simulink library "bh_6dof_LIBRARY"  (R2016a)
settings: Solver=VariableStepAuto  StartTime=0.0  StopTime=10.0  RelTol=1e-3
undefined symbols (not defined in the file): mot_1_volts, mot_2_volts, mot_3_volts, mot_4_volts, P_veh
libraries: simulink_extras x3, bh_6dof_LIBRARY x1
settings Model: Creator=bhorton  LastModifiedBy=bhorton
settings DataIOCC: LimitDataPoints=on
settings DebuggingCC: AllowSymbolicDim=off
settings ModelReferenceCC: PropagateSignalLabelsOutOfModel=off
settings GRTTargetCC: GeneratePreprocessorConditionals=Use local settings

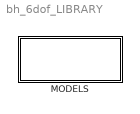
== system bh_6dof_LIBRARY ==
  MODELS : Subsystem

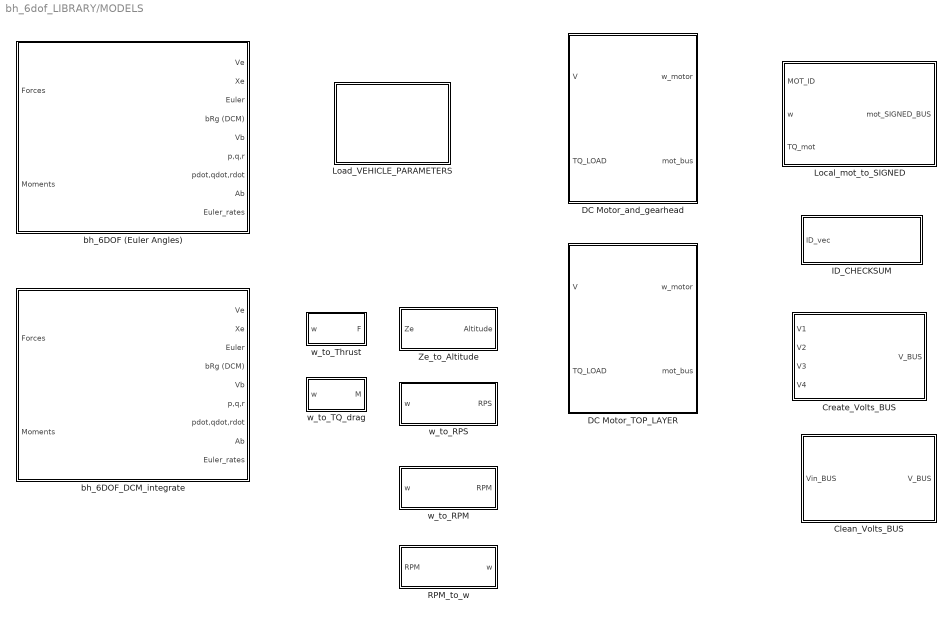
== system bh_6dof_LIBRARY/MODELS ==
  Clean_Volts_BUS : Subsystem  mask{v_min=0, v_max=7}
      mask prompts: v_min "V minimun (volts)"; v_max "V maximum (volts)"
      mask Display: fprintf('CLEAN \n\n VOLTS BUS \n\n Vmin = %.2f \n Vmax = %.2f',v_min, v_max);
  Create_Volts_BUS : Subsystem  mask{v_min=0, v_max=7}
      mask prompts: v_min "V minimun (volts)"; v_max "V maximum (volts)"
      mask Display: fprintf('VOLTS BUS \n\n Vmin = %.2f \n Vmax = %.2f',v_min, v_max);
  DC Motor_TOP_LAYER : Subsystem  mask(DC motor){P_mot_S=struct('ID',0,'Ka',1,'b',1,'I',1,'R',1,'L',1,'Ke',1)}
      mask prompts: P_mot_S "Enter your MOTOR param STRUCT"
      mask help: DC motor
      mask DialogControl Container9 Prompt: Tab
      mask Display: fprintf('DC motor\n\nID= %d',P_mot_S.ID)
  DC Motor_and_gearhead : Subsystem  mask(DC motor){K=1, B=1e-6, J=1e-7, GearRatio=1, R=1, L=1, Kb=1, ID=1}
      mask prompts: K "Torque constant (N.m/A)"; B "Viscous friction co-efficient (N.m.s)"; J "Rotor Inertia (kg.m^2)"; GearRatio "Gear ratio (w_motor/w_wheel)"; R "Armature resistance (ohms)"; L "Armature Inductance (Henry)"; Kb "Back Emf constant (V.sec/rad)"; ID "Motor_ID  (#1 to #4)"
      mask help: DC motor
      mask Display: disp('DC motor')
  ID_CHECKSUM : Subsystem
      mask Display: fprintf('ID\nChecksum')
  Load_VEHICLE_PARAMETERS : Subsystem
      settings: OpenFcn=bh_quad_params
      mask Display: disp('Double click\nto\nLOAD\nvehicle \n parameters')
  Local_mot_to_SIGNED : Subsystem
  RPM_to_w : Subsystem
      mask Display: fprintf('RPM\nto\nw(rad/sec)')
  Ze_to_Altitude : Subsystem
      mask Display: fprintf('Ze \n to \n ALTITUDE');
  bh_6DOF (Euler Angles) : Subsystem  mask(bh_6DOF EoM (Body Axis)){inertia_0=P_veh.I, mass_0=P_veh.mass, xme_0=P_veh.Xe_init, Vm_0=P_veh.Vb_init, pm_0=P_veh.wb_init, eul_0=P_veh.eul_init}
      mask prompts: inertia_0 "Vehicle Inertia, [kg.m^2]"; mass_0 "Vehicle Mass, [kg]"; xme_0 "Initial position in inertial axes [Xe,Ye,Ze], [m]"; Vm_0 "Initial velocity in body axes [U,v,w], [m/sec]"; pm_0 "Initial body rotation rates [p,q,r], [rad/sec]"; eul_0 "Initial Euler orientation [yaw, pitch, roll], [rad]"
      mask DialogControl DescTextVar Prompt: Implementation of a 6-DOF rigid body equations of motion.
      mask DialogControl Control16 Prompt: Euler angles are used to describe angular pose.
      mask DialogControl Control22 Prompt: The co-ordinate transformation that converts the components of a
      mask DialogControl Control23 Prompt: G-frame vector into its components in the B-frame, is:
      mask DialogControl Control24 Prompt: vb = pR3X(psi) * pR2Y(theta) * pR1Z(phi) * vg
      mask DialogControl Control25 Prompt: vb = bRg * vg
      mask DialogControl Control53 Prompt: You can READ more about PASSIVE rotations, HERE.
      mask DialogControl Control53 Callback: winopen('CONCEPT_PASSIVE_rotations.pdf')
      mask DialogControl Control26 Prompt: To actively reposition (ie: rotate) a B-frame that is initially coincident
      mask DialogControl Control27 Prompt: with the inertial G-frame, into a new pose, we would:
      mask DialogControl Control28 Prompt: vg = inv(pR1Z(phi)) * inv(pR2Y(theta)) * inv(pR3X(psi)) * vb
      mask DialogControl Control30 Prompt: If we define:    aR( ) == inv( pR()  ),  then we can write the above as:
      mask DialogControl Control32 Prompt: vg = aR1Z(phi) * aR2Y(theta) * aR3(psi) * vb
      mask DialogControl Control40 Prompt: You can READ more about ACTIVE rotations, HERE.
      mask DialogControl Control40 Callback: winopen('CONCEPT_ACTIVE_rotations.pdf')
      mask DialogControl Control11 Prompt: ATTENTION:  note the order of the angles in the list above.
      mask DialogControl Control12 Prompt: This is DIFFERENT to the order used in the Aerospace blockset.
      mask DialogControl Control6 Prompt: In this EULER angle implementation we define the
      mask DialogControl Control7 Prompt: following sequence that rotates a G-frame
      mask DialogControl Control8 Prompt: into a B-frame:
      mask DialogControl Control9_copy Prompt: 1.)  R1Z  : a local rotation about the Z axis by phi, (YAW)
      mask DialogControl Control9_copy_copy Prompt: 2.)  R2Y  : a local rotation about the Y axis by theta, (PITCH)
      mask DialogControl Control17 Prompt: 3.)  R3X  : a local rotation about the X axis by psi, (ROLL)
      mask DialogControl Control18 Prompt: The translational Rigid body Equations of motion are:
      mask DialogControl Control20 Prompt: The rotational Rigid body Equations of motion are
      mask Display:
      | port_label('input',1,'{{Fb_{xyz}} (N)}','texmode','on');
      | port_label('input',2,'{{Mb_{xyz}} (N-m)}','texmode','on');
      | port_label('output',1,'{V_e (m/s)}','texmode','on');
      | port_label('output',2,'{X_e (m)}','texmode','on');
      | port_label('output',3,'{\Phi_{Z1} \theta_{Y2} \Psi_{X3} (rad)}','texmode','on');
      | port_label('output',4,'{DCM bRg }','texmode','on');
      | port_label('output',5,'{V_b (m/s)}','texmode','on');
      | port_label('output',6,'{{\omega_b (rad/s)}}','texmode','on');
      | port_label('output',7,'{{d\omega_b/dt}}','texmode','on');
      | port_label('output',8,'{A_b (m/s^2)}','texmode','on');
      | port_label('output',9,'{d\Phi_{Z1} d\theta_{Y2} d\Psi_{X3} (rad/sec)}','texmode','on');
      | 
      | text(0.5,0.7248,'Body\nEuler Angles','horizontalAlignment','center')
      | text(0.5,0.3112,'Fixed\nMass','horizontalAlignment','center')
  bh_6DOF_DCM_integrate : Subsystem  mask(bh_6DOF EoM (Body Axis) DCM approach){inertia_0=P_veh.I, mass_0=P_veh.mass, xme_0=P_veh.Xe_init, Vm_0=P_veh.Vb_init, pm_0=P_veh.wb_init, eul_0=P_veh.eul_init}
      mask prompts: inertia_0 "Vehicle Inertia, [kg.m^2]"; mass_0 "Vehicle Mass, [kg]"; xme_0 "Initial position in inertial axes [Xe,Ye,Ze], [m]"; Vm_0 "Initial velocity in body axes [U,v,w], [m/sec]"; pm_0 "Initial body rotation rates [p,q,r], [rad/sec]"; eul_0 "Initial Euler orientation [yaw, pitch, roll], [rad]"
      mask DialogControl DescTextVar Prompt: Implementation of a 6-DOF rigid body equations of motion.
      mask DialogControl Control16 Prompt: Euler angles are used to describe angular pose. We integrate the DCM derivative to calculate the Euler angles.
      mask DialogControl Control22 Prompt: The co-ordinate transformation that converts the components of a
      mask DialogControl Control23 Prompt: G-frame vector into its components in the B-frame, is:
      mask DialogControl Control24 Prompt: vb = pR3X(psi) * pR2Y(theta) * pR1Z(phi) * vg
      mask DialogControl Control25 Prompt: vb = bRg * vg
      mask DialogControl Control53 Prompt: You can READ more about PASSIVE rotations, HERE.
      mask DialogControl Control53 Callback: winopen('CONCEPT_PASSIVE_rotations.pdf')
      mask DialogControl Control26 Prompt: To actively reposition (ie: rotate) a B-frame that is initially coincident
      mask DialogControl Control27 Prompt: with the inertial G-frame, into a new pose, we would:
      mask DialogControl Control28 Prompt: vg = inv(pR1Z(phi)) * inv(pR2Y(theta)) * inv(pR3X(psi)) * vb
      mask DialogControl Control30 Prompt: If we define:    aR( ) == inv( pR()  ),  then we can write the above as:
      mask DialogControl Control32 Prompt: vg = aR1Z(phi) * aR2Y(theta) * aR3(psi) * vb
      mask DialogControl Control40 Prompt: You can READ more about ACTIVE rotations, HERE.
      mask DialogControl Control40 Callback: winopen('CONCEPT_ACTIVE_rotations.pdf')
      mask DialogControl Control11 Prompt: ATTENTION:  note the order of the angles in the list above.
      mask DialogControl Control12 Prompt: This is DIFFERENT to the order used in the Aerospace blockset.
      mask DialogControl Control6 Prompt: In this EULER angle implementation we define the
      mask DialogControl Control7 Prompt: following sequence that rotates a G-frame
      mask DialogControl Control8 Prompt: into a B-frame:
      mask DialogControl Control9_copy Prompt: 1.)  R1Z  : a local rotation about the Z axis by phi, (YAW)
      mask DialogControl Control9_copy_copy Prompt: 2.)  R2Y  : a local rotation about the Y axis by theta, (PITCH)
      mask DialogControl Control17 Prompt: 3.)  R3X  : a local rotation about the X axis by psi, (ROLL)
      mask DialogControl Control18 Prompt: The translational Rigid body Equations of motion are:
      mask DialogControl Control20 Prompt: The rotational Rigid body Equations of motion are
      mask Display:
      | port_label('input',1,'{{Fb_{xyz}} (N)}','texmode','on');
      | port_label('input',2,'{{Mb_{xyz}} (N-m)}','texmode','on');
      | port_label('output',1,'{V_e (m/s)}','texmode','on');
      | port_label('output',2,'{X_e (m)}','texmode','on');
      | port_label('output',3,'{\Phi_{Z1} \theta_{Y2} \Psi_{X3} (rad)}','texmode','on');
      | port_label('output',4,'{DCM bRg }','texmode','on');
      | port_label('output',5,'{V_b (m/s)}','texmode','on');
      | port_label('output',6,'{{\omega_b (rad/s)}}','texmode','on');
      | port_label('output',7,'{{d\omega_b/dt}}','texmode','on');
      | port_label('output',8,'{A_b (m/s^2)}','texmode','on');
      | port_label('output',9,'{d\Phi_{Z1} d\theta_{Y2} d\Psi_{X3} (rad/sec)}','texmode','on');
      | 
      | text(0.5,0.7248,'DCM\nintegration','horizontalAlignment','center')
      | 
      | text(0.5,0.3112,'Fixed\nMass','horizontalAlignment','center')
  w_to_RPM : Subsystem
      mask Display: fprintf('w(rad/sec)\nto\nRPM')
  w_to_RPS : Subsystem
      mask Display: fprintf('w(rad/sec)\nto\nRPS')
  w_to_TQ_drag : Subsystem  mask(w_to_TQdrag){k=0}
      mask prompts: k "k (N/ ( rad/sec)^2 )"
      mask help:
      | Convert angular speed w(rad/sec) into drag TORQUE,  M (N.m).
      | A simple quadratic rule is used:
      |
      | M = k * w^2
      settings: AttributesFormatString=k = %<k>
  w_to_Thrust : Subsystem  mask(w_to_thrust){k=0}
      mask prompts: k "k (N/ ( rad/sec)^2 )"
      mask help:
      | Convert angular speed w(rad/sec) into lift thrust F (N).
      | A simple quadratic rule is used:
      |
      | F = k * w^2
      settings: AttributesFormatString=k = %<k>

== system bh_6dof_LIBRARY/MODELS/Clean_Volts_BUS ==
  Vin_BUS : Inport
  Bus Assignment : BusAssignment  AssignedSignals=mot_1_volts,mot_2_volts,mot_3_volts,mot_4_volts
  Bus Selector : BusSelector  OutputSignals=mot_1_volts,mot_2_volts,mot_3_volts,mot_4_volts
  Saturation{4..7} (4 alike) : Saturate  UpperLimit=v_max  LowerLimit=v_min
  V_BUS : Outport
  wires:
  Bus Selector/1 -> Saturation4/1  "<mot_1_volts>"
  Bus Selector/2 -> Saturation5/1  "<mot_2_volts>"
  Bus Selector/3 -> Saturation6/1  "<mot_3_volts>"
  Bus Selector/4 -> Saturation7/1  "<mot_4_volts>"
  Vin_BUS/1 -> Bus Assignment/1, Bus Selector/1
  Saturation4/1 -> Bus Assignment/2
  Saturation7/1 -> Bus Assignment/5
  Saturation6/1 -> Bus Assignment/4
  Saturation5/1 -> Bus Assignment/3
  Bus Assignment/1 -> V_BUS/1

== system bh_6dof_LIBRARY/MODELS/Create_Volts_BUS ==
  V1 : Inport
  V2 : Inport  Port=2
  V3 : Inport  Port=3
  V4 : Inport  Port=4
  Bus Creator : BusCreator  Inputs=4
  Saturation{,1..3} (4 alike) : Saturate  UpperLimit=v_max  LowerLimit=v_min
  V_BUS : Outport
  wires:
  Bus Creator/1 -> V_BUS/1
  Saturation/1 -> Bus Creator/1  "mot_1_volts"
  Saturation3/1 -> Bus Creator/4  "mot_4_volts"
  Saturation2/1 -> Bus Creator/3  "mot_3_volts"
  Saturation1/1 -> Bus Creator/2  "mot_2_volts"
  V1/1 -> Saturation/1
  V2/1 -> Saturation1/1
  V3/1 -> Saturation2/1
  V4/1 -> Saturation3/1

== system bh_6dof_LIBRARY/MODELS/DC Motor_TOP_LAYER ==
  V : Inport
  TQ_LOAD : Inport  Port=2
  DC Motor_and_gearhead : bh_6dof_LIBRARY/MODELS/DC Motor_and_gearhead  K=P_mot_S.Ka  B=P_mot_S.b  J=P_mot_S.I  R=P_mot_S.R  L=P_mot_S.L  Kb=P_mot_S.Ke  ID=P_mot_S.ID
  w_motor : Outport
  mot_bus : Outport  Port=2
  wires:
  DC Motor_and_gearhead/2 -> mot_bus/1
  DC Motor_and_gearhead/1 -> w_motor/1
  TQ_LOAD/1 -> DC Motor_and_gearhead/2
  V/1 -> DC Motor_and_gearhead/1

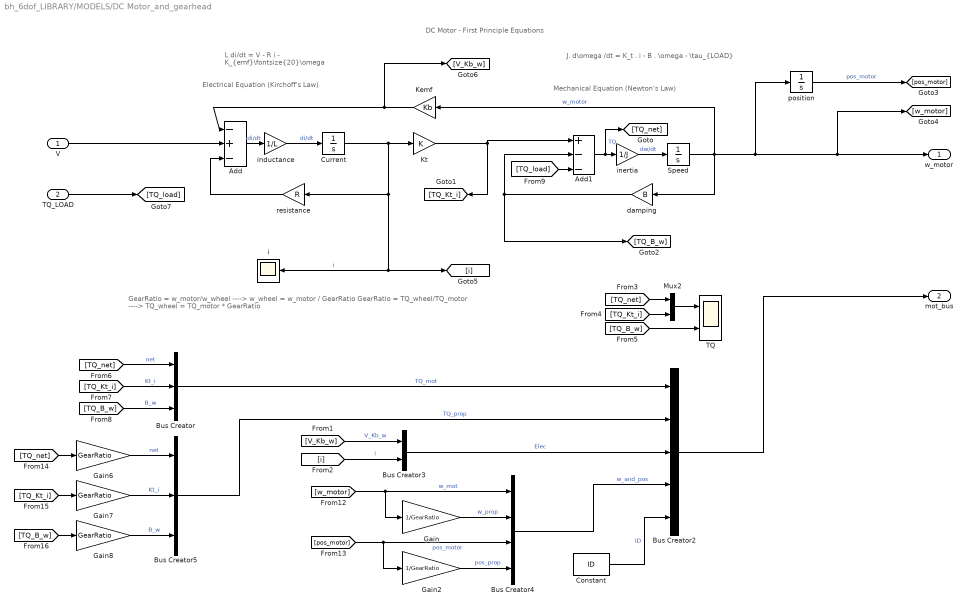
== system bh_6dof_LIBRARY/MODELS/DC Motor_and_gearhead ==
  note: GearRatio = w_motor/w_wheel    ---->   w_wheel = w_motor / GearRatio
      |
      | GearRatio = TQ_wheel/TQ_motor  ---->  TQ_wheel = TQ_motor * GearRatio
  note: Mechanical Equation
      | (Newton's Law)
  note: L di/dt = V - R i - K_{emf}\fontsize{20}\omega
  note: J. d\omega /dt = K_t . i - B . \omega - \tau_{LOAD}
  note: DC Motor - First Principle Equations
  note: Electrical Equation
      | (Kirchoff's Law)
  V : Inport
  TQ_LOAD : Inport  Port=2
  Add : Sum  Inputs=-+-
  Add1 : Sum  Inputs=+--
  Bus Creator : BusCreator  Inputs=3
  Bus Creator2 : BusCreator  Inputs=5
  Bus Creator3 : BusCreator  Inputs=2
  Bus Creator4 : BusCreator  Inputs=4
  Bus Creator5 : BusCreator  Inputs=3
  Constant : Constant  Value=ID
  Current : Integrator
  Gain : Gain  Gain=1/GearRatio
  Gain2 : Gain  Gain=1/GearRatio
  Gain6 : Gain  Gain=GearRatio
  Gain7 : Gain  Gain=GearRatio
  Gain8 : Gain  Gain=GearRatio
  Kemf : Gain  Gain=Kb
  Kt : Gain  Gain=K
  Mux2 : Mux  Inputs=2
  Speed : Integrator
  TQ : Scope  NumInputPorts=2
  damping : Gain  Gain=B
  i : Scope
  inductance : Gain  Gain=1/L
  inertia : Gain  Gain=1/J
  position : Integrator
  resistance : Gain  Gain=R
  w_motor : Outport
  mot_bus : Outport  Port=2
  wires:
  inertia/1 -> Speed/1  "dw/dt"
  damping/1 -> [TQ_B_w], Add1/2
  Kt/1 -> Add1/1, [TQ_Kt_i]
  inductance/1 -> Current/1  "di/dt"
  Speed/1 -> Kemf/1, position/1, [w_motor], w_motor/1, damping/1  "w_motor"
  Add1/1 -> [TQ_net], inertia/1  "TQ"
  Current/1 -> Kt/1, resistance/1, [i], i/1  "i"
  Add/1 -> inductance/1  "di/dt"
  resistance/1 -> Add/3
  Kemf/1 -> [V_Kb_w], Add/1
  position/1 -> [pos_motor]  "pos_motor"
  Mux2/1 -> TQ/1
  [TQ_net] -> Mux2/1
  [TQ_Kt_i] -> Mux2/2
  [TQ_B_w] -> TQ/2
  [TQ_net] -> Bus Creator/1  "net"
  [TQ_B_w] -> Bus Creator/3  "B_w"
  [TQ_Kt_i] -> Bus Creator/2  "Kt_i"
  Bus Creator/1 -> Bus Creator2/1  "TQ_mot"
  [i] -> Bus Creator3/2  "i"
  [V_Kb_w] -> Bus Creator3/1  "V_Kb_w"
  [w_motor] -> Gain/1, Bus Creator4/1  "w_mot"
  Gain/1 -> Bus Creator4/2  "w_prop"
  [pos_motor] -> Gain2/1, Bus Creator4/3  "pos_motor"
  Gain2/1 -> Bus Creator4/4  "pos_prop"
  Bus Creator5/1 -> Bus Creator2/2  "TQ_prop"
  Bus Creator4/1 -> Bus Creator2/4  "w_and_pos"
  Bus Creator3/1 -> Bus Creator2/3  "Elec"
  Bus Creator2/1 -> mot_bus/1
  [TQ_net] -> Gain6/1
  Gain6/1 -> Bus Creator5/1  "net"
  Gain8/1 -> Bus Creator5/3  "B_w"
  Gain7/1 -> Bus Creator5/2  "Kt_i"
  [TQ_Kt_i] -> Gain7/1
  [TQ_B_w] -> Gain8/1
  TQ_LOAD/1 -> [TQ_load]
  [TQ_load] -> Add1/3
  V/1 -> Add/2
  Constant/1 -> Bus Creator2/5  "ID"

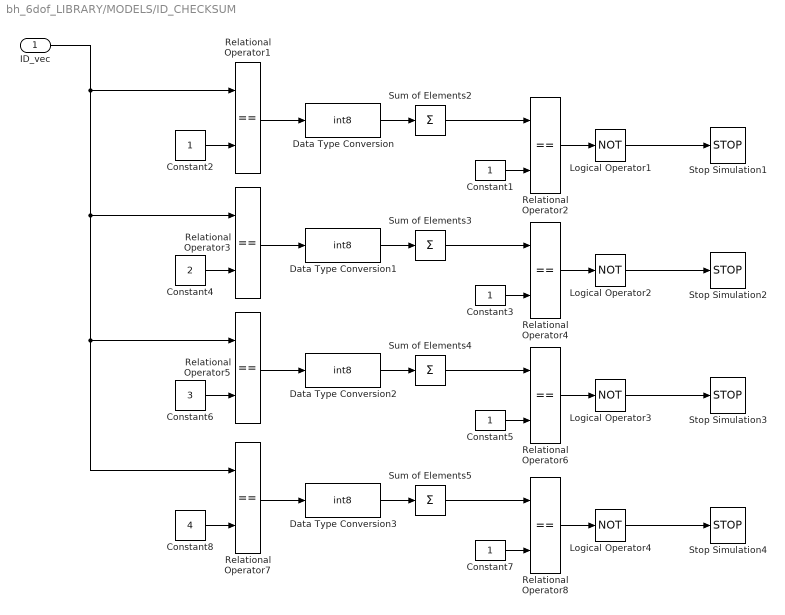
== system bh_6dof_LIBRARY/MODELS/ID_CHECKSUM ==
  ID_vec : Inport
  Constant{1..3,5,7} (5 alike) : Constant
  Constant4 : Constant  Value=2
  Constant6 : Constant  Value=3
  Constant8 : Constant  Value=4
  Data Type Conversion{,1..3} (4 alike) : DataTypeConversion  OutDataTypeStr=int8
  Logical Operator{1..4} (4 alike) : Logic  Operator=NOT  AllPortsSameDT=off  OutDataTypeStr=boolean
  Relational Operator{1..8} (8 alike) : RelationalOperator  Operator===  OutDataTypeStr=boolean
  Stop Simulation{1..4} (4 alike) : Stop
  Sum of Elements{2..5} (4 alike) : Sum  Inputs=+
  wires:
  Relational Operator1/1 -> Data Type Conversion/1
  Data Type Conversion/1 -> Sum of Elements2/1
  Sum of Elements2/1 -> Relational Operator2/1
  Constant1/1 -> Relational Operator2/2
  Relational Operator2/1 -> Logical Operator1/1
  Constant2/1 -> Relational Operator1/2
  Logical Operator1/1 -> Stop Simulation1/1
  Relational Operator3/1 -> Data Type Conversion1/1
  Data Type Conversion1/1 -> Sum of Elements3/1
  Sum of Elements3/1 -> Relational Operator4/1
  Constant3/1 -> Relational Operator4/2
  Relational Operator4/1 -> Logical Operator2/1
  Constant4/1 -> Relational Operator3/2
  Logical Operator2/1 -> Stop Simulation2/1
  Relational Operator5/1 -> Data Type Conversion2/1
  Data Type Conversion2/1 -> Sum of Elements4/1
  Sum of Elements4/1 -> Relational Operator6/1
  Constant5/1 -> Relational Operator6/2
  Relational Operator6/1 -> Logical Operator3/1
  Constant6/1 -> Relational Operator5/2
  Logical Operator3/1 -> Stop Simulation3/1
  ID_vec/1 -> Relational Operator7/1, Relational Operator5/1, Relational Operator3/1, Relational Operator1/1
  Relational Operator7/1 -> Data Type Conversion3/1
  Data Type Conversion3/1 -> Sum of Elements5/1
  Sum of Elements5/1 -> Relational Operator8/1
  Constant7/1 -> Relational Operator8/2
  Relational Operator8/1 -> Logical Operator4/1
  Constant8/1 -> Relational Operator7/2
  Logical Operator4/1 -> Stop Simulation4/1

== system bh_6dof_LIBRARY/MODELS/Load_VEHICLE_PARAMETERS ==

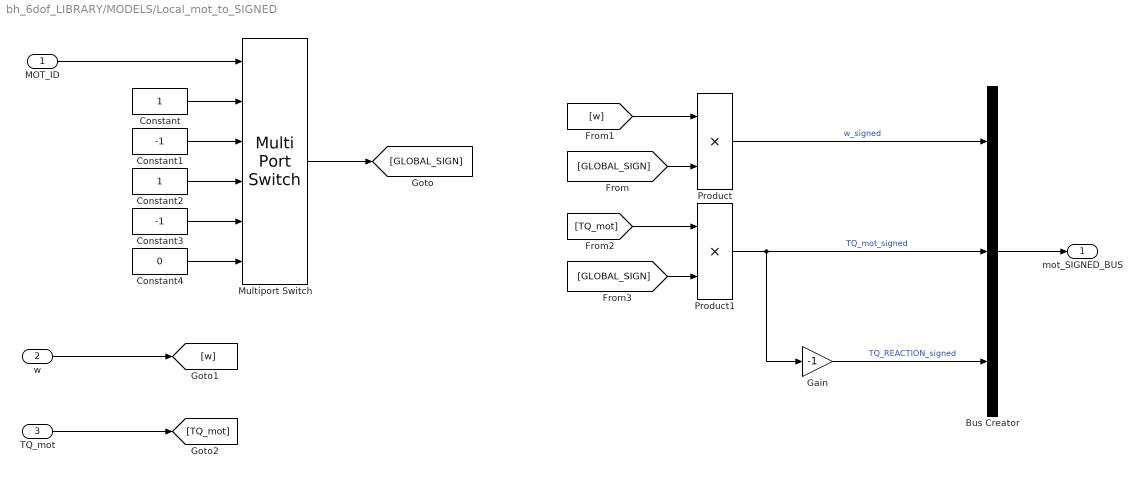
== system bh_6dof_LIBRARY/MODELS/Local_mot_to_SIGNED ==
  MOT_ID : Inport
  w : Inport  Port=2
  TQ_mot : Inport  Port=3
  Bus Creator : BusCreator  Inputs=3
  Constant : Constant
  Constant1 : Constant  Value=-1
  Constant2 : Constant
  Constant3 : Constant  Value=-1
  Constant4 : Constant  Value=0
  Gain : Gain  Gain=-1
  Multiport Switch : MultiPortSwitch  Inputs=4  DataPortForDefault=Additional data port
  Product : Product
  Product1 : Product
  mot_SIGNED_BUS : Outport
  wires:
  Constant1/1 -> Multiport Switch/3
  Constant/1 -> Multiport Switch/2
  Constant3/1 -> Multiport Switch/5
  Constant4/1 -> Multiport Switch/6
  MOT_ID/1 -> Multiport Switch/1
  Constant2/1 -> Multiport Switch/4
  Multiport Switch/1 -> [GLOBAL_SIGN]
  TQ_mot/1 -> [TQ_mot]
  w/1 -> [w]
  [GLOBAL_SIGN] -> Product/2
  [w] -> Product/1
  Product/1 -> Bus Creator/1  "w_signed"
  [GLOBAL_SIGN] -> Product1/2
  [TQ_mot] -> Product1/1
  Product1/1 -> Bus Creator/2, Gain/1  "TQ_mot_signed"
  Gain/1 -> Bus Creator/3  "TQ_REACTION_signed"
  Bus Creator/1 -> mot_SIGNED_BUS/1

== system bh_6dof_LIBRARY/MODELS/RPM_to_w ==
  RPM : Inport
  Constant : Constant  Value=3.141592653589793
  Constant1 : Constant  Value=60
  Gain1 : Gain  Gain=2
  Product : Product
  Product1 : Product  Inputs=*/
  w : Outport
  wires:
  Product1/1 -> Product/1  "RPS"
  Constant1/1 -> Product1/2
  RPM/1 -> Product1/1  "RPM"
  Constant/1 -> Gain1/1
  Gain1/1 -> Product/2  "2PI"
  Product/1 -> w/1  "w_rad_per_sec"

== system bh_6dof_LIBRARY/MODELS/Ze_to_Altitude ==
  Ze : Inport
  Altitude : Outport
  wires:
  Ze/1 -> Altitude/1

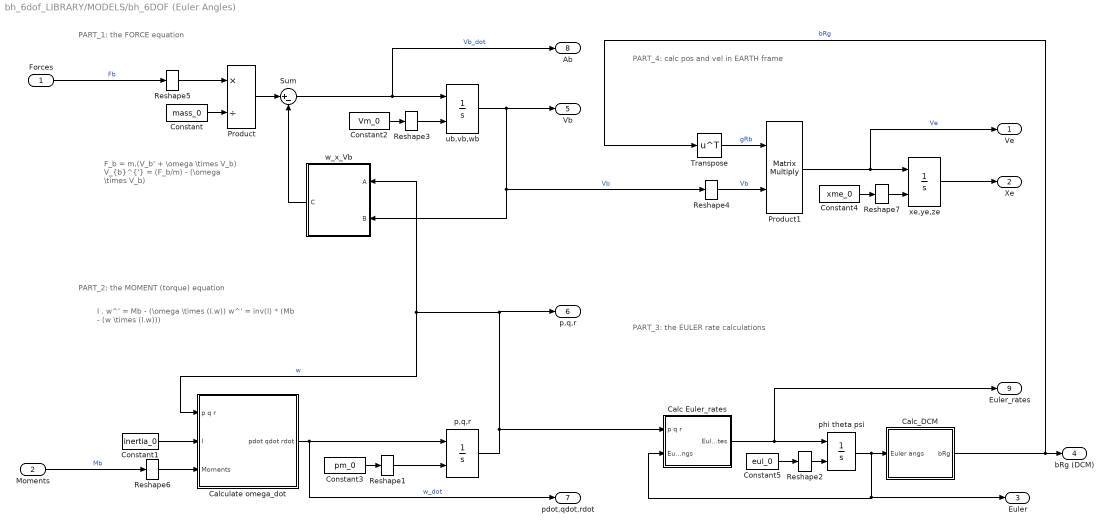
== system bh_6dof_LIBRARY/MODELS/bh_6DOF (Euler Angles) ==
  note: PART_4: calc pos and vel in EARTH frame
  note: PART_3: the EULER rate calculations
  note: PART_2: the MOMENT (torque) equation
  note: PART_1: the FORCE equation
  note: F_b = m.(V_b' + \omega \times V_b)
      |
      | V_{b}^{'} = (F_b/m) - (\omega \times V_b)
  note: I . w^' = Mb - (\omega \times (I.w))
      |
      | w^' = inv(I) * (Mb - (w \times (I.w)))
  Forces : Inport
  Moments : Inport  Port=2
  Calc Euler_rates : Subsystem
  Calc_DCM : Subsystem
  Calculate omega_dot : Subsystem
  Constant : Constant  Value=mass_0  OutDataTypeStr=Inherit: Inherit via back propagation
  Constant1 : Constant  Value=inertia_0  OutDataTypeStr=Inherit: Inherit via back propagation
  Constant2 : Constant  Value=Vm_0  OutDataTypeStr=Inherit: Inherit via back propagation
  Constant3 : Constant  Value=pm_0  OutDataTypeStr=Inherit: Inherit via back propagation
  Constant4 : Constant  Value=xme_0  OutDataTypeStr=Inherit: Inherit via back propagation
  Constant5 : Constant  Value=eul_0  OutDataTypeStr=Inherit: Inherit via back propagation
  Product : Product  Inputs=*/  SaturateOnIntegerOverflow=on  OutDataTypeStr=Inherit: Same as first input
  Product1 : Product  Multiplication=Matrix(*)  SaturateOnIntegerOverflow=on  InputSameDT=on  OutDataTypeStr=Inherit: Same as first input
  Reshape{1..7} (7 alike) : Reshape  OutputDimensionality=Column vector (2-D)
  Sum : Sum  Inputs=|+-  SaturateOnIntegerOverflow=on
  Transpose : Math  Operator=transpose  SaturateOnIntegerOverflow=on
  "p,q,r " : Integrator  InitialConditionSource=external  InitialCondition=pm_0
  phi theta psi : Integrator  InitialConditionSource=external  InitialCondition=eul_0
  ub,vb,wb : Integrator  InitialConditionSource=external  InitialCondition=Vm_0
  w_x_Vb : Subsystem
      mask Display:
      | text(.5,.5,'Cross\nProduct\n\nC = AxB', ...
      | 	'HorizontalAlignment','Center',...
      | 	'VerticalAlignment','middle')
  xe,ye,ze : Integrator  InitialConditionSource=external  InitialCondition=xme_0
  Ve : Outport
  Xe : Outport  Port=2
  Euler : Outport  Port=3
  bRg (DCM) : Outport  Port=4
  Vb : Outport  Port=5
  p,q,r : Outport  Port=6
  pdot,qdot,rdot : Outport  Port=7
  Ab : Outport  Port=8
  Euler_rates : Outport  Port=9
  wires:
  Constant4/1 -> Reshape7/1
  Reshape7/1 -> xe,ye,ze/2
  Product1/1 -> xe,ye,ze/1, Ve/1  "Ve"
  Constant3/1 -> Reshape1/1
  Reshape1/1 -> "p,q,r "/2
  Reshape6/1 -> Calculate omega_dot/3(Moments)
  Reshape5/1 -> Product/1
  Reshape3/1 -> ub,vb,wb/2
  Constant2/1 -> Reshape3/1
  Calculate omega_dot/1(pdot qdot rdot) -> "p,q,r "/1, pdot,qdot,rdot/1  "w_dot"
  Reshape4/1 -> Product1/2  "Vb"
  Transpose/1 -> Product1/1  "gRb"
  Constant1/1 -> Calculate omega_dot/2(I)
  w_x_Vb/1(C) -> Sum/2
  xe,ye,ze/1 -> Xe/1
  "p,q,r "/1 -> w_x_Vb/1(A), Calculate omega_dot/1(p q r), p,q,r/1, Calc Euler_rates/1("p q r ")  "w"
  Moments/1 -> Reshape6/1  "Mb"
  Product/1 -> Sum/1
  Constant/1 -> Product/2
  Forces/1 -> Reshape5/1  "Fb"
  ub,vb,wb/1 -> Vb/1, w_x_Vb/2(B), Reshape4/1  "Vb"
  Sum/1 -> ub,vb,wb/1, Ab/1  "Vb_dot"
  Constant5/1 -> Reshape2/1
  Reshape2/1 -> phi theta psi/2
  Calc Euler_rates/1(Euler_rates) -> Euler_rates/1, phi theta psi/1
  phi theta psi/1 -> Calc_DCM/1(Euler angs), Euler/1, Calc Euler_rates/2(Euler_angs)
  Calc_DCM/1(bRg) -> Transpose/1, bRg (DCM)/1  "bRg"

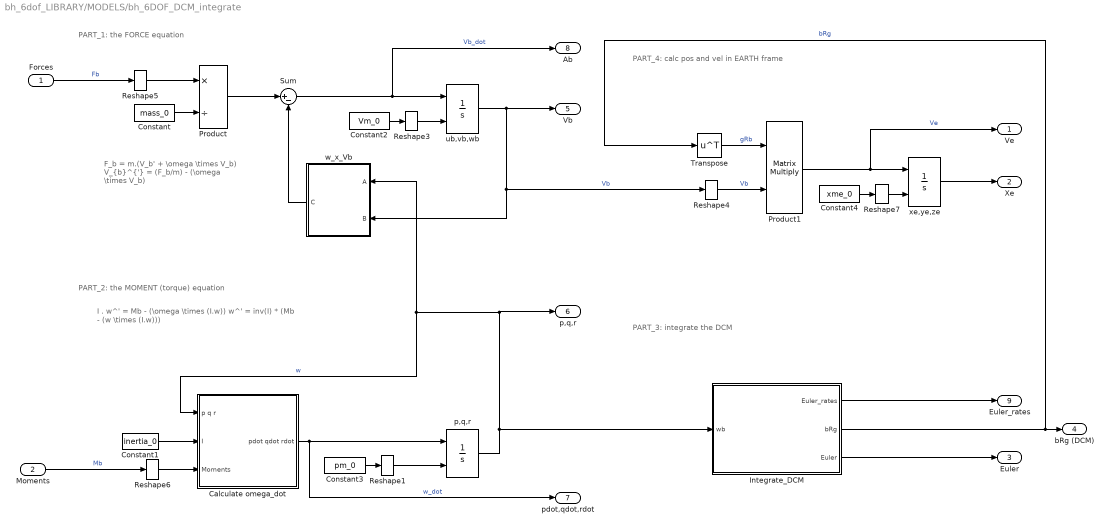
== system bh_6dof_LIBRARY/MODELS/bh_6DOF_DCM_integrate ==
  note: I . w^' = Mb - (\omega \times (I.w))
      |
      | w^' = inv(I) * (Mb - (w \times (I.w)))
  note: F_b = m.(V_b' + \omega \times V_b)
      |
      | V_{b}^{'} = (F_b/m) - (\omega \times V_b)
  note: PART_1: the FORCE equation
  note: PART_2: the MOMENT (torque) equation
  note: PART_3: integrate the DCM
  note: PART_4: calc pos and vel in EARTH frame
  Forces : Inport
  Moments : Inport  Port=2
  Calculate omega_dot : Subsystem
  Constant : Constant  Value=mass_0  OutDataTypeStr=Inherit: Inherit via back propagation
  Constant1 : Constant  Value=inertia_0  OutDataTypeStr=Inherit: Inherit via back propagation
  Constant2 : Constant  Value=Vm_0  OutDataTypeStr=Inherit: Inherit via back propagation
  Constant3 : Constant  Value=pm_0  OutDataTypeStr=Inherit: Inherit via back propagation
  Constant4 : Constant  Value=xme_0  OutDataTypeStr=Inherit: Inherit via back propagation
  Integrate_DCM : Subsystem
  Product : Product  Inputs=*/  SaturateOnIntegerOverflow=on  OutDataTypeStr=Inherit: Same as first input
  Product1 : Product  Multiplication=Matrix(*)  SaturateOnIntegerOverflow=on  InputSameDT=on  OutDataTypeStr=Inherit: Same as first input
  Reshape{1,3..7} (6 alike) : Reshape  OutputDimensionality=Column vector (2-D)
  Sum : Sum  Inputs=|+-  SaturateOnIntegerOverflow=on
  Transpose : Math  Operator=transpose  SaturateOnIntegerOverflow=on
  "p,q,r " : Integrator  InitialConditionSource=external  InitialCondition=pm_0
  ub,vb,wb : Integrator  InitialConditionSource=external  InitialCondition=Vm_0
  w_x_Vb : Subsystem
      mask Display:
      | text(.5,.5,'Cross\nProduct\n\nC = AxB', ...
      | 	'HorizontalAlignment','Center',...
      | 	'VerticalAlignment','middle')
  xe,ye,ze : Integrator  InitialConditionSource=external  InitialCondition=xme_0
  Ve : Outport
  Xe : Outport  Port=2
  Euler : Outport  Port=3
  bRg (DCM) : Outport  Port=4
  Vb : Outport  Port=5
  p,q,r : Outport  Port=6
  pdot,qdot,rdot : Outport  Port=7
  Ab : Outport  Port=8
  Euler_rates : Outport  Port=9
  wires:
  Integrate_DCM/2(bRg) -> Transpose/1, bRg (DCM)/1  "bRg"
  Sum/1 -> Ab/1, ub,vb,wb/1  "Vb_dot"
  ub,vb,wb/1 -> Reshape4/1, w_x_Vb/2(B), Vb/1  "Vb"
  Forces/1 -> Reshape5/1  "Fb"
  Constant/1 -> Product/2
  Product/1 -> Sum/1
  Moments/1 -> Reshape6/1  "Mb"
  "p,q,r "/1 -> Integrate_DCM/1(wb), p,q,r/1, Calculate omega_dot/1(p q r), w_x_Vb/1(A)  "w"
  xe,ye,ze/1 -> Xe/1
  w_x_Vb/1(C) -> Sum/2
  Constant1/1 -> Calculate omega_dot/2(I)
  Transpose/1 -> Product1/1  "gRb"
  Reshape4/1 -> Product1/2  "Vb"
  Calculate omega_dot/1(pdot qdot rdot) -> pdot,qdot,rdot/1, "p,q,r "/1  "w_dot"
  Constant2/1 -> Reshape3/1
  Reshape3/1 -> ub,vb,wb/2
  Reshape5/1 -> Product/1
  Reshape6/1 -> Calculate omega_dot/3(Moments)
  Reshape1/1 -> "p,q,r "/2
  Constant3/1 -> Reshape1/1
  Product1/1 -> Ve/1, xe,ye,ze/1  "Ve"
  Reshape7/1 -> xe,ye,ze/2
  Constant4/1 -> Reshape7/1
  Integrate_DCM/1(Euler_rates) -> Euler_rates/1
  Integrate_DCM/3(Euler) -> Euler/1

== system bh_6dof_LIBRARY/MODELS/w_to_RPM ==
  w : Inport
  Constant : Constant  Value=3.141592653589793
  Gain : Gain  Gain=60
  Gain1 : Gain  Gain=2
  Product : Product  Inputs=*/
  RPM : Outport
  wires:
  w/1 -> Gain/1  "w_per_sec"
  Gain/1 -> Product/1  "w_per_min"
  Constant/1 -> Gain1/1
  Gain1/1 -> Product/2  "2PI"
  Product/1 -> RPM/1

== system bh_6dof_LIBRARY/MODELS/w_to_RPS ==
  w : Inport
  Constant : Constant  Value=3.141592653589793
  Gain1 : Gain  Gain=2
  Product : Product  Inputs=*/
  RPS : Outport
  wires:
  w/1 -> Product/1  "w_per_sec"
  Constant/1 -> Gain1/1
  Gain1/1 -> Product/2  "2PI"
  Product/1 -> RPS/1

== system bh_6dof_LIBRARY/MODELS/w_to_TQ_drag ==
  w : Inport
  Gain2 : Gain  Gain=k
  Math Function1 : Math  Operator=square  SaturateOnIntegerOverflow=on
  M : Outport
  wires:
  Gain2/1 -> M/1
  Math Function1/1 -> Gain2/1
  w/1 -> Math Function1/1

== system bh_6dof_LIBRARY/MODELS/w_to_Thrust ==
  w : Inport
  Gain2 : Gain  Gain=k
  Math Function1 : Math  Operator=square  SaturateOnIntegerOverflow=on
  F : Outport
  wires:
  Gain2/1 -> F/1
  Math Function1/1 -> Gain2/1
  w/1 -> Math Function1/1

== system bh_6dof_LIBRARY/MODELS/bh_6DOF (Euler Angles)/Calc Euler_rates ==
  "p q r " : Inport
  Euler_angs : Inport  Port=2
  Demux1 : Demux  Outputs=3
  Demux2 : Demux  Outputs=3
  Demux3 : Demux  Outputs=3
  Mux1 : Mux  Inputs=3
  Reshape1 : Reshape  OutputDimensionality=Column vector (2-D)
  Reshape2 : Reshape  OutputDimensionality=Column vector (2-D)
  Terminator : Terminator
  my_euler_rates : MATLAB Function  TreatAsAtomicUnit=on
  Euler_rates : Outport
  wires:
  Demux1/3 -> my_euler_rates/2(psi)  "psi"
  Demux1/1 -> Terminator/1  "phi"
  Demux1/2 -> my_euler_rates/1(theta)  "theta"
  "p q r "/1 -> Reshape1/1
  Euler_angs/1 -> Demux1/1
  Demux3/1 -> my_euler_rates/3(p)
  Demux3/2 -> my_euler_rates/4(q)
  Demux3/3 -> my_euler_rates/5(r)
  Mux1/1 -> Reshape2/1
  Reshape2/1 -> Euler_rates/1
  Demux2/1 -> Mux1/1  "phidot_Z1_yaw"
  Demux2/2 -> Mux1/2  "thetadot_Y2_pitch"
  Demux2/3 -> Mux1/3  "psidot_X3_roll"
  my_euler_rates/1(euler_rates) -> Demux2/1  "euler_rates"
  Reshape1/1 -> Demux3/1  "wb"

== system bh_6dof_LIBRARY/MODELS/bh_6DOF (Euler Angles)/Calc_DCM ==
  Euler angs : Inport
  Demux3 : Demux  Outputs=3
  calc_DCM : MATLAB Function  TreatAsAtomicUnit=on
  bRg : Outport
  wires:
  Euler angs/1 -> Demux3/1
  Demux3/1 -> calc_DCM/1(phi)  "phi"
  Demux3/2 -> calc_DCM/2(theta)  "thetsa"
  Demux3/3 -> calc_DCM/3(psi)  "psi"
  calc_DCM/1(bRg) -> bRg/1

== system bh_6dof_LIBRARY/MODELS/bh_6DOF (Euler Angles)/Calculate omega_dot ==
  note: I . w^' = Mb - (\omega \times (I.w))
      |
      | w^' = inv(I) * (Mb - (w \times (I.w)))
  p q r : Inport
  I : Inport  Port=2
  Moments : Inport  Port=3
  Product : Product  Multiplication=Matrix(*)  SaturateOnIntegerOverflow=on  InputSameDT=on  OutDataTypeStr=Inherit: Same as first input
  Product1 : Product  Inputs=/  Multiplication=Matrix(*)  SaturateOnIntegerOverflow=on  OutDataTypeStr=Inherit: Same as first input
  Product2 : Product  Multiplication=Matrix(*)  SaturateOnIntegerOverflow=on  OutDataTypeStr=Inherit: Same as first input
  Reshape2 : Reshape  OutputDimensionality=Column vector (2-D)
  Reshape3 : Reshape  OutputDimensionality=Column vector (2-D)
  Reshape4 : Reshape  OutputDimensionality=Column vector (2-D)
  Sum2 : Sum  Inputs=+|-  SaturateOnIntegerOverflow=on
  w_x_(I.w) : Subsystem
      mask Display:
      | text(.5,.5,'Cross\nProduct\n\nC = AxB', ...
      | 	'HorizontalAlignment','Center',...
      | 	'VerticalAlignment','middle')
  pdot qdot rdot : Outport
  wires:
  Product2/1 -> pdot qdot rdot/1  "w_dot"
  Sum2/1 -> Product2/2  "Mb - (w x (I.w))"
  Product1/1 -> Product2/1  "inv(I)"
  [I] -> Product1/1
  Reshape4/1 -> Sum2/2  "w x (I.w)"
  Reshape3/1 -> Sum2/1  "Mb"
  Product/1 -> w_x_(I.w)/2(B)  "I.w"
  p q r/1 -> Reshape2/1
  [I] -> Product/1  "I"
  Reshape2/1 -> Product/2, w_x_(I.w)/1(A)  "w"
  I/1 -> [I]  "I"
  Moments/1 -> Reshape3/1
  w_x_(I.w)/1(C) -> Reshape4/1

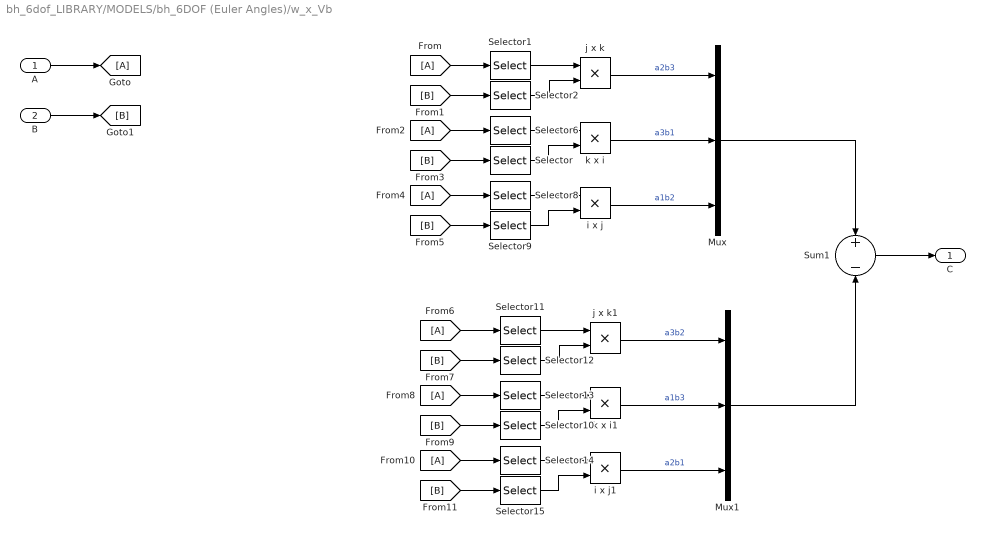
== system bh_6dof_LIBRARY/MODELS/bh_6DOF (Euler Angles)/w_x_Vb ==
  A : Inport
  B : Inport  Port=2
  Mux : Mux  Inputs=3
  Mux1 : Mux  Inputs=3
  Selector{,8,13,15} (4 alike) : Selector  InputPortWidth=3  IndexOptions=Index vector (dialog)  Indices=1  OutputSizes=1
  Selector{1,9,12,14} (4 alike) : Selector  InputPortWidth=3  IndexOptions=Index vector (dialog)  Indices=2  OutputSizes=1
  Selector{2,6,10..11} (4 alike) : Selector  InputPortWidth=3  IndexOptions=Index vector (dialog)  Indices=3  OutputSizes=1
  Sum1 : Sum  Inputs=+|-  SaturateOnIntegerOverflow=on  InputSameDT=on  OutDataTypeStr=Inherit: Same as first input
  i x j : Product  SaturateOnIntegerOverflow=on  InputSameDT=on  OutDataTypeStr=Inherit: Same as first input
  i x j1 : Product  SaturateOnIntegerOverflow=on  InputSameDT=on  OutDataTypeStr=Inherit: Same as first input
  j x k : Product  SaturateOnIntegerOverflow=on  InputSameDT=on  OutDataTypeStr=Inherit: Same as first input
  j x k1 : Product  SaturateOnIntegerOverflow=on  InputSameDT=on  OutDataTypeStr=Inherit: Same as first input
  k x i : Product  SaturateOnIntegerOverflow=on  InputSameDT=on  OutDataTypeStr=Inherit: Same as first input
  k x i1 : Product  SaturateOnIntegerOverflow=on  InputSameDT=on  OutDataTypeStr=Inherit: Same as first input
  C : Outport
  wires:
  Selector15/1 -> i x j1/2
  Selector14/1 -> i x j1/1
  [B] -> Selector15/1
  [A] -> Selector14/1
  Selector10/1 -> k x i1/2
  Selector13/1 -> k x i1/1
  [B] -> Selector10/1
  [A] -> Selector13/1
  [A] -> Selector11/1
  [B] -> Selector12/1
  Selector12/1 -> j x k1/2
  Selector11/1 -> j x k1/1
  Mux1/1 -> Sum1/2
  j x k1/1 -> Mux1/1  "a3b2"
  k x i1/1 -> Mux1/2  "a1b3"
  i x j1/1 -> Mux1/3  "a2b1"
  Selector9/1 -> i x j/2
  Selector8/1 -> i x j/1
  [B] -> Selector9/1
  [A] -> Selector8/1
  Selector/1 -> k x i/2
  Selector6/1 -> k x i/1
  [B] -> Selector/1
  [A] -> Selector6/1
  [A] -> Selector1/1
  [B] -> Selector2/1
  A/1 -> [A]
  B/1 -> [B]
  Selector2/1 -> j x k/2
  Selector1/1 -> j x k/1
  Sum1/1 -> C/1
  Mux/1 -> Sum1/1
  j x k/1 -> Mux/1  "a2b3"
  k x i/1 -> Mux/2  "a3b1"
  i x j/1 -> Mux/3  "a1b2"

== system bh_6dof_LIBRARY/MODELS/bh_6DOF_DCM_integrate/Calculate omega_dot ==
  note: I . w^' = Mb - (\omega \times (I.w))
      |
      | w^' = inv(I) * (Mb - (w \times (I.w)))
  p q r : Inport
  I : Inport  Port=2
  Moments : Inport  Port=3
  Product : Product  Multiplication=Matrix(*)  SaturateOnIntegerOverflow=on  InputSameDT=on  OutDataTypeStr=Inherit: Same as first input
  Product1 : Product  Inputs=/  Multiplication=Matrix(*)  SaturateOnIntegerOverflow=on  OutDataTypeStr=Inherit: Same as first input
  Product2 : Product  Multiplication=Matrix(*)  SaturateOnIntegerOverflow=on  OutDataTypeStr=Inherit: Same as first input
  Reshape2 : Reshape  OutputDimensionality=Column vector (2-D)
  Reshape3 : Reshape  OutputDimensionality=Column vector (2-D)
  Reshape4 : Reshape  OutputDimensionality=Column vector (2-D)
  Sum2 : Sum  Inputs=+|-  SaturateOnIntegerOverflow=on
  w_x_(I.w) : Subsystem
      mask Display:
      | text(.5,.5,'Cross\nProduct\n\nC = AxB', ...
      | 	'HorizontalAlignment','Center',...
      | 	'VerticalAlignment','middle')
  pdot qdot rdot : Outport
  wires:
  w_x_(I.w)/1(C) -> Reshape4/1
  Moments/1 -> Reshape3/1
  I/1 -> [I]  "I"
  Reshape2/1 -> w_x_(I.w)/1(A), Product/2  "w"
  [I] -> Product/1  "I"
  p q r/1 -> Reshape2/1
  Product/1 -> w_x_(I.w)/2(B)  "I.w"
  Reshape3/1 -> Sum2/1  "Mb"
  Reshape4/1 -> Sum2/2  "w x (I.w)"
  [I] -> Product1/1
  Product1/1 -> Product2/1  "inv(I)"
  Sum2/1 -> Product2/2  "Mb - (w x (I.w))"
  Product2/1 -> pdot qdot rdot/1  "w_dot"

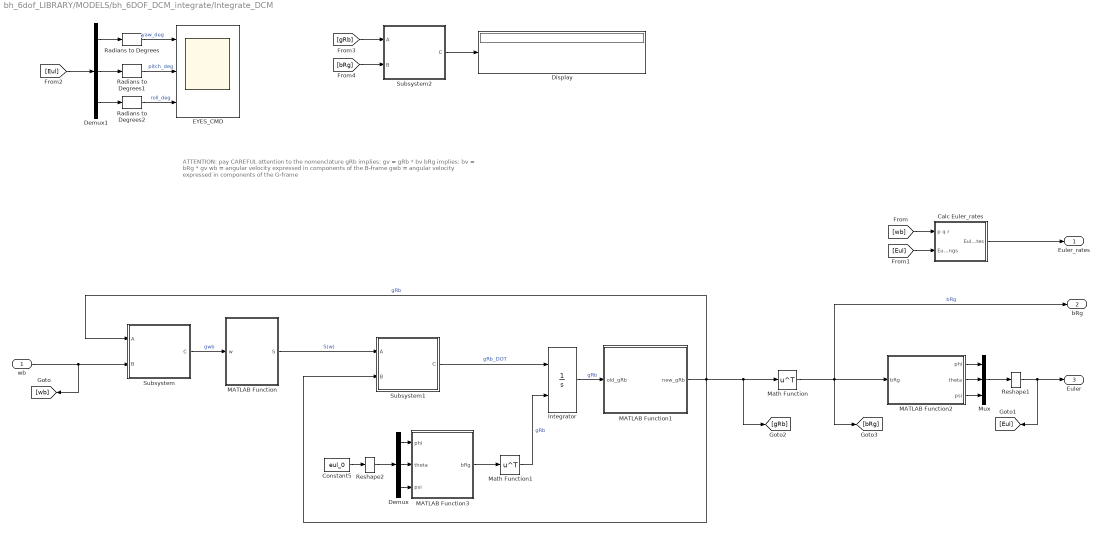
== system bh_6dof_LIBRARY/MODELS/bh_6DOF_DCM_integrate/Integrate_DCM ==
  note: ATTENTION: pay CAREFUL attention to the nomenclature
      | gRb implies: gv = gRb * bv
      | bRg implies: bv = bRg * gv
      |
      | wb = angular velocity expressed in components of the B-frame
      | gwb = angular velocity expressed in components of the G-frame
  wb : Inport
  Calc Euler_rates : Subsystem
  Constant5 : Constant  Value=eul_0  OutDataTypeStr=Inherit: Inherit via back propagation
  Demux : Demux  Outputs=3
  Demux1 : Demux  Outputs=3
  Display : Display
  EYES_CMD : Scope  NumInputPorts=3
  Integrator : Integrator  InitialConditionSource=external
  MATLAB Function : MATLAB Function  TreatAsAtomicUnit=on
  MATLAB Function1 : MATLAB Function  TreatAsAtomicUnit=on
  MATLAB Function2 : MATLAB Function  TreatAsAtomicUnit=on
  MATLAB Function3 : MATLAB Function  TreatAsAtomicUnit=on
  Math Function : Math  Operator=transpose  SaturateOnIntegerOverflow=on
  Math Function1 : Math  Operator=transpose  SaturateOnIntegerOverflow=on
  Mux : Mux  Inputs=3
  Radians to Degrees : simulink_extras/Transformations/Radians to Degrees
  Radians to Degrees1 : simulink_extras/Transformations/Radians to Degrees
  Radians to Degrees2 : simulink_extras/Transformations/Radians to Degrees
  Reshape1 : Reshape  OutputDimensionality=Column vector (2-D)
  Reshape2 : Reshape  OutputDimensionality=Column vector (2-D)
  Subsystem : Subsystem
      mask Display: disp('A * B')
  Subsystem1 : Subsystem
      mask Display: disp('A * B')
  Subsystem2 : Subsystem
      mask Display: disp('A * B')
  Euler_rates : Outport
  bRg : Outport  Port=2
  Euler : Outport  Port=3
  wires:
  MATLAB Function/1(S) -> Subsystem1/1(A)  "S(w)"
  Math Function/1 -> MATLAB Function2/1(bRg), bRg/1, [bRg]  "bRg"
  Integrator/1 -> MATLAB Function1/1(old_gRb)  "gRb"
  Subsystem1/1(C) -> Integrator/1  "gRb_DOT"
  MATLAB Function2/1(phi) -> Mux/1
  MATLAB Function2/2(theta) -> Mux/2
  MATLAB Function2/3(psi) -> Mux/3
  wb/1 -> Subsystem/2(B), [wb]
  Demux/3 -> MATLAB Function3/3(psi)
  Math Function1/1 -> Integrator/2  "gRb"
  Demux/1 -> MATLAB Function3/1(phi)
  Demux/2 -> MATLAB Function3/2(theta)
  MATLAB Function3/1(bRg) -> Math Function1/1
  Constant5/1 -> Reshape2/1
  Reshape2/1 -> Demux/1
  Mux/1 -> Reshape1/1
  Reshape1/1 -> Euler/1, [Eul]
  [wb] -> Calc Euler_rates/1("p q r ")
  [Eul] -> Calc Euler_rates/2(Euler_angs)
  Subsystem2/1(C) -> Display/1
  Demux1/1 -> Radians to Degrees/1
  Radians to Degrees/1 -> EYES_CMD/1  "yaw_deg"
  Radians to Degrees1/1 -> EYES_CMD/2  "pitch_deg"
  Radians to Degrees2/1 -> EYES_CMD/3  "roll_deg"
  Demux1/3 -> Radians to Degrees2/1
  Demux1/2 -> Radians to Degrees1/1
  [Eul] -> Demux1/1
  Calc Euler_rates/1(Euler_rates) -> Euler_rates/1
  Subsystem/1(C) -> MATLAB Function/1(w)  "gwb"
  [gRb] -> Subsystem2/1(A)
  [bRg] -> Subsystem2/2(B)
  MATLAB Function1/1(new_gRb) -> Subsystem1/2(B), Subsystem/1(A), [gRb], Math Function/1  "gRb"

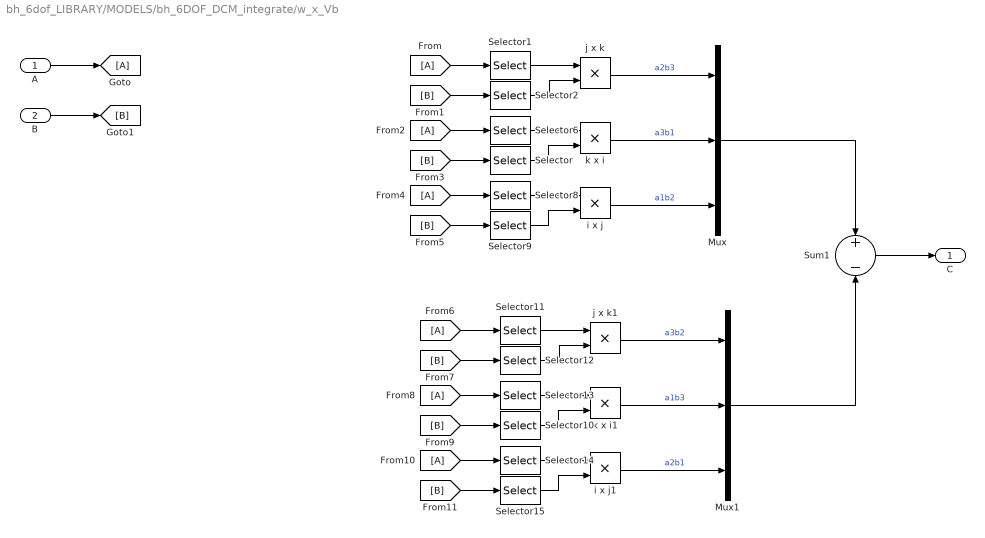
== system bh_6dof_LIBRARY/MODELS/bh_6DOF_DCM_integrate/w_x_Vb ==
  A : Inport
  B : Inport  Port=2
  Mux : Mux  Inputs=3
  Mux1 : Mux  Inputs=3
  Selector{,8,13,15} (4 alike) : Selector  InputPortWidth=3  IndexOptions=Index vector (dialog)  Indices=1  OutputSizes=1
  Selector{1,9,12,14} (4 alike) : Selector  InputPortWidth=3  IndexOptions=Index vector (dialog)  Indices=2  OutputSizes=1
  Selector{2,6,10..11} (4 alike) : Selector  InputPortWidth=3  IndexOptions=Index vector (dialog)  Indices=3  OutputSizes=1
  Sum1 : Sum  Inputs=+|-  SaturateOnIntegerOverflow=on  InputSameDT=on  OutDataTypeStr=Inherit: Same as first input
  i x j : Product  SaturateOnIntegerOverflow=on  InputSameDT=on  OutDataTypeStr=Inherit: Same as first input
  i x j1 : Product  SaturateOnIntegerOverflow=on  InputSameDT=on  OutDataTypeStr=Inherit: Same as first input
  j x k : Product  SaturateOnIntegerOverflow=on  InputSameDT=on  OutDataTypeStr=Inherit: Same as first input
  j x k1 : Product  SaturateOnIntegerOverflow=on  InputSameDT=on  OutDataTypeStr=Inherit: Same as first input
  k x i : Product  SaturateOnIntegerOverflow=on  InputSameDT=on  OutDataTypeStr=Inherit: Same as first input
  k x i1 : Product  SaturateOnIntegerOverflow=on  InputSameDT=on  OutDataTypeStr=Inherit: Same as first input
  C : Outport
  wires:
  i x j/1 -> Mux/3  "a1b2"
  k x i/1 -> Mux/2  "a3b1"
  j x k/1 -> Mux/1  "a2b3"
  Mux/1 -> Sum1/1
  Sum1/1 -> C/1
  Selector1/1 -> j x k/1
  Selector2/1 -> j x k/2
  B/1 -> [B]
  A/1 -> [A]
  [B] -> Selector2/1
  [A] -> Selector1/1
  [A] -> Selector6/1
  [B] -> Selector/1
  Selector6/1 -> k x i/1
  Selector/1 -> k x i/2
  [A] -> Selector8/1
  [B] -> Selector9/1
  Selector8/1 -> i x j/1
  Selector9/1 -> i x j/2
  i x j1/1 -> Mux1/3  "a2b1"
  k x i1/1 -> Mux1/2  "a1b3"
  j x k1/1 -> Mux1/1  "a3b2"
  Mux1/1 -> Sum1/2
  Selector11/1 -> j x k1/1
  Selector12/1 -> j x k1/2
  [B] -> Selector12/1
  [A] -> Selector11/1
  [A] -> Selector13/1
  [B] -> Selector10/1
  Selector13/1 -> k x i1/1
  Selector10/1 -> k x i1/2
  [A] -> Selector14/1
  [B] -> Selector15/1
  Selector14/1 -> i x j1/1
  Selector15/1 -> i x j1/2

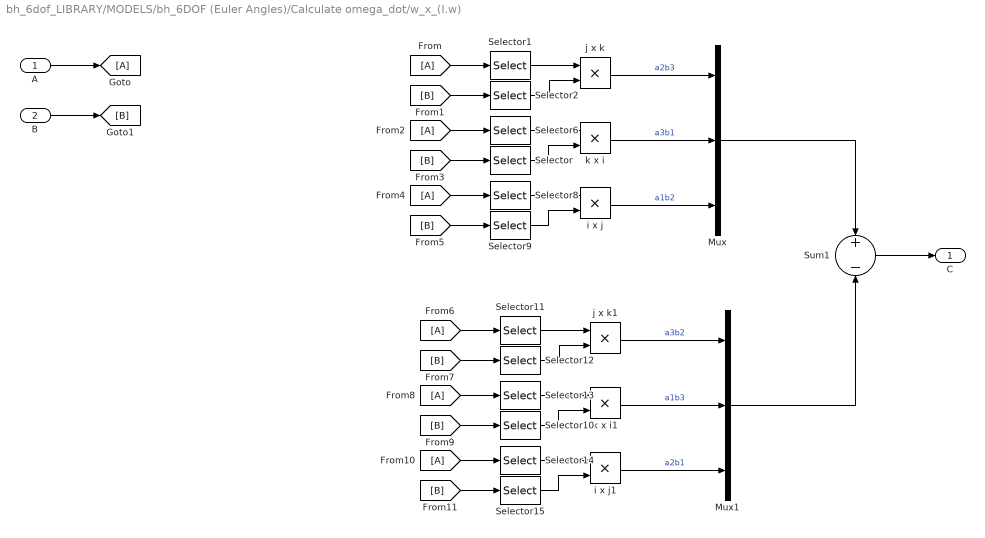
== system bh_6dof_LIBRARY/MODELS/bh_6DOF (Euler Angles)/Calculate omega_dot/w_x_(I.w) ==
  A : Inport
  B : Inport  Port=2
  Mux : Mux  Inputs=3
  Mux1 : Mux  Inputs=3
  Selector{,8,13,15} (4 alike) : Selector  InputPortWidth=3  IndexOptions=Index vector (dialog)  Indices=1  OutputSizes=1
  Selector{1,9,12,14} (4 alike) : Selector  InputPortWidth=3  IndexOptions=Index vector (dialog)  Indices=2  OutputSizes=1
  Selector{2,6,10..11} (4 alike) : Selector  InputPortWidth=3  IndexOptions=Index vector (dialog)  Indices=3  OutputSizes=1
  Sum1 : Sum  Inputs=+|-  SaturateOnIntegerOverflow=on  InputSameDT=on  OutDataTypeStr=Inherit: Same as first input
  i x j : Product  SaturateOnIntegerOverflow=on  InputSameDT=on  OutDataTypeStr=Inherit: Same as first input
  i x j1 : Product  SaturateOnIntegerOverflow=on  InputSameDT=on  OutDataTypeStr=Inherit: Same as first input
  j x k : Product  SaturateOnIntegerOverflow=on  InputSameDT=on  OutDataTypeStr=Inherit: Same as first input
  j x k1 : Product  SaturateOnIntegerOverflow=on  InputSameDT=on  OutDataTypeStr=Inherit: Same as first input
  k x i : Product  SaturateOnIntegerOverflow=on  InputSameDT=on  OutDataTypeStr=Inherit: Same as first input
  k x i1 : Product  SaturateOnIntegerOverflow=on  InputSameDT=on  OutDataTypeStr=Inherit: Same as first input
  C : Outport
  wires:
  Selector15/1 -> i x j1/2
  Selector14/1 -> i x j1/1
  [B] -> Selector15/1
  [A] -> Selector14/1
  Selector10/1 -> k x i1/2
  Selector13/1 -> k x i1/1
  [B] -> Selector10/1
  [A] -> Selector13/1
  [A] -> Selector11/1
  [B] -> Selector12/1
  Selector12/1 -> j x k1/2
  Selector11/1 -> j x k1/1
  Mux1/1 -> Sum1/2
  j x k1/1 -> Mux1/1  "a3b2"
  k x i1/1 -> Mux1/2  "a1b3"
  i x j1/1 -> Mux1/3  "a2b1"
  Selector9/1 -> i x j/2
  Selector8/1 -> i x j/1
  [B] -> Selector9/1
  [A] -> Selector8/1
  Selector/1 -> k x i/2
  Selector6/1 -> k x i/1
  [B] -> Selector/1
  [A] -> Selector6/1
  [A] -> Selector1/1
  [B] -> Selector2/1
  A/1 -> [A]
  B/1 -> [B]
  Selector2/1 -> j x k/2
  Selector1/1 -> j x k/1
  Sum1/1 -> C/1
  Mux/1 -> Sum1/1
  j x k/1 -> Mux/1  "a2b3"
  k x i/1 -> Mux/2  "a3b1"
  i x j/1 -> Mux/3  "a1b2"

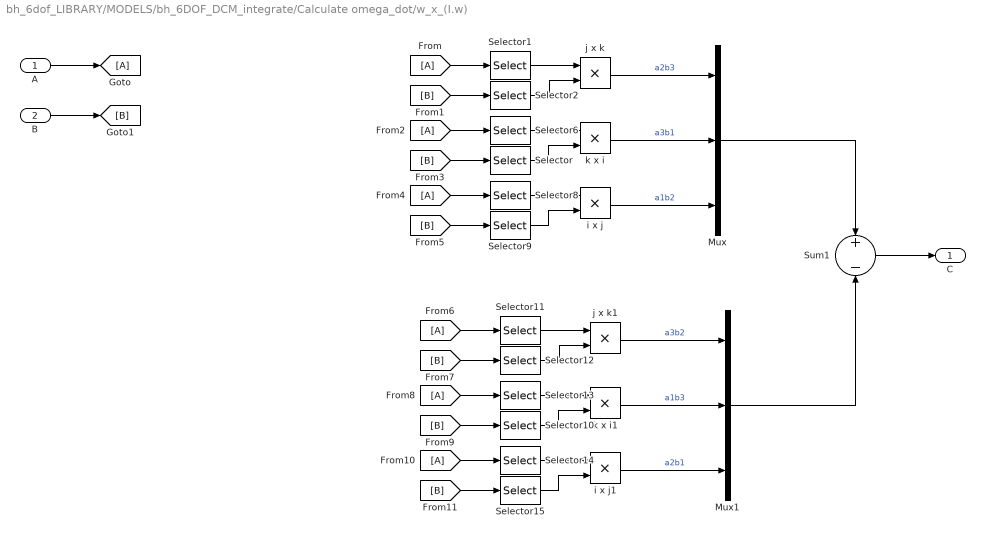
== system bh_6dof_LIBRARY/MODELS/bh_6DOF_DCM_integrate/Calculate omega_dot/w_x_(I.w) ==
  A : Inport
  B : Inport  Port=2
  Mux : Mux  Inputs=3
  Mux1 : Mux  Inputs=3
  Selector{,8,13,15} (4 alike) : Selector  InputPortWidth=3  IndexOptions=Index vector (dialog)  Indices=1  OutputSizes=1
  Selector{1,9,12,14} (4 alike) : Selector  InputPortWidth=3  IndexOptions=Index vector (dialog)  Indices=2  OutputSizes=1
  Selector{2,6,10..11} (4 alike) : Selector  InputPortWidth=3  IndexOptions=Index vector (dialog)  Indices=3  OutputSizes=1
  Sum1 : Sum  Inputs=+|-  SaturateOnIntegerOverflow=on  InputSameDT=on  OutDataTypeStr=Inherit: Same as first input
  i x j : Product  SaturateOnIntegerOverflow=on  InputSameDT=on  OutDataTypeStr=Inherit: Same as first input
  i x j1 : Product  SaturateOnIntegerOverflow=on  InputSameDT=on  OutDataTypeStr=Inherit: Same as first input
  j x k : Product  SaturateOnIntegerOverflow=on  InputSameDT=on  OutDataTypeStr=Inherit: Same as first input
  j x k1 : Product  SaturateOnIntegerOverflow=on  InputSameDT=on  OutDataTypeStr=Inherit: Same as first input
  k x i : Product  SaturateOnIntegerOverflow=on  InputSameDT=on  OutDataTypeStr=Inherit: Same as first input
  k x i1 : Product  SaturateOnIntegerOverflow=on  InputSameDT=on  OutDataTypeStr=Inherit: Same as first input
  C : Outport
  wires:
  i x j/1 -> Mux/3  "a1b2"
  k x i/1 -> Mux/2  "a3b1"
  j x k/1 -> Mux/1  "a2b3"
  Mux/1 -> Sum1/1
  Sum1/1 -> C/1
  Selector1/1 -> j x k/1
  Selector2/1 -> j x k/2
  B/1 -> [B]
  A/1 -> [A]
  [B] -> Selector2/1
  [A] -> Selector1/1
  [A] -> Selector6/1
  [B] -> Selector/1
  Selector6/1 -> k x i/1
  Selector/1 -> k x i/2
  [A] -> Selector8/1
  [B] -> Selector9/1
  Selector8/1 -> i x j/1
  Selector9/1 -> i x j/2
  i x j1/1 -> Mux1/3  "a2b1"
  k x i1/1 -> Mux1/2  "a1b3"
  j x k1/1 -> Mux1/1  "a3b2"
  Mux1/1 -> Sum1/2
  Selector11/1 -> j x k1/1
  Selector12/1 -> j x k1/2
  [B] -> Selector12/1
  [A] -> Selector11/1
  [A] -> Selector13/1
  [B] -> Selector10/1
  Selector13/1 -> k x i1/1
  Selector10/1 -> k x i1/2
  [A] -> Selector14/1
  [B] -> Selector15/1
  Selector14/1 -> i x j1/1
  Selector15/1 -> i x j1/2

== system bh_6dof_LIBRARY/MODELS/bh_6DOF_DCM_integrate/Integrate_DCM/Calc Euler_rates ==
  "p q r " : Inport
  Euler_angs : Inport  Port=2
  Demux1 : Demux  Outputs=3
  Demux2 : Demux  Outputs=3
  Demux3 : Demux  Outputs=3
  Mux1 : Mux  Inputs=3
  Reshape1 : Reshape  OutputDimensionality=Column vector (2-D)
  Reshape2 : Reshape  OutputDimensionality=Column vector (2-D)
  Terminator : Terminator
  my_euler_rates : MATLAB Function  TreatAsAtomicUnit=on
  Euler_rates : Outport
  wires:
  Reshape1/1 -> Demux3/1  "wb"
  my_euler_rates/1(euler_rates) -> Demux2/1  "euler_rates"
  Demux2/3 -> Mux1/3  "psidot_X3_roll"
  Demux2/2 -> Mux1/2  "thetadot_Y2_pitch"
  Demux2/1 -> Mux1/1  "phidot_Z1_yaw"
  Reshape2/1 -> Euler_rates/1
  Mux1/1 -> Reshape2/1
  Demux3/3 -> my_euler_rates/5(r)
  Demux3/2 -> my_euler_rates/4(q)
  Demux3/1 -> my_euler_rates/3(p)
  Euler_angs/1 -> Demux1/1
  "p q r "/1 -> Reshape1/1
  Demux1/2 -> my_euler_rates/1(theta)  "theta"
  Demux1/1 -> Terminator/1  "phi"
  Demux1/3 -> my_euler_rates/2(psi)  "psi"

== system bh_6dof_LIBRARY/MODELS/bh_6DOF_DCM_integrate/Integrate_DCM/Subsystem ==
  note: C = A * B
  A : Inport
  B : Inport  Port=2
  Product2 : Product  Multiplication=Matrix(*)
  C : Outport
  wires:
  B/1 -> Product2/2
  A/1 -> Product2/1
  Product2/1 -> C/1

== system bh_6dof_LIBRARY/MODELS/bh_6DOF_DCM_integrate/Integrate_DCM/Subsystem1 ==
  note: C = A * B
  A : Inport
  B : Inport  Port=2
  Product2 : Product  Multiplication=Matrix(*)
  C : Outport
  wires:
  B/1 -> Product2/2
  A/1 -> Product2/1
  Product2/1 -> C/1

== system bh_6dof_LIBRARY/MODELS/bh_6DOF_DCM_integrate/Integrate_DCM/Subsystem2 ==
  note: C = A * B
  A : Inport
  B : Inport  Port=2
  Product2 : Product  Multiplication=Matrix(*)
  C : Outport
  wires:
  B/1 -> Product2/2
  A/1 -> Product2/1
  Product2/1 -> C/1

== matlab function bh_6dof_LIBRARY/MODELS/bh_6DOF_DCM_integrate/Integrate_DCM/Calc Euler_rates/my_euler_rates ==
  data: theta input; euler_rates output; psi input; p input; q input; r input
function euler_rates = my_euler_rates(theta,psi,p,q,r)
%#codegen

%    This function was generated by the Symbolic Math Toolbox version 7.0.
%    09-Jun-2016 10:28:25

euler_rates = [(r.*cos(psi)+q.*sin(psi))./cos(theta);
                q.*cos(psi)-r.*sin(psi);
               (p.*cos(theta)+r.*cos(psi).*sin(theta)+q.*sin(psi).*sin(theta))./cos(theta)];

== matlab function bh_6dof_LIBRARY/MODELS/bh_6DOF (Euler Angles)/Calc Euler_rates/my_euler_rates ==
  data: theta input; euler_rates output; psi input; p input; q input; r input
function euler_rates = my_euler_rates(theta,psi,p,q,r)
%#codegen

%    This function was generated by the Symbolic Math Toolbox version 7.0.
%    09-Jun-2016 10:28:25

euler_rates = [(r.*cos(psi)+q.*sin(psi))./cos(theta);
                q.*cos(psi)-r.*sin(psi);
               (p.*cos(theta)+r.*cos(psi).*sin(theta)+q.*sin(psi).*sin(theta))./cos(theta)];

== matlab function bh_6dof_LIBRARY/MODELS/bh_6DOF_DCM_integrate/Integrate_DCM/MATLAB Function1 ==
  data: old_gRb input; new_gRb output
function new_gRb = correct_gRb(old_gRb)
%#codegen

% The correction technique implementde here is the one described by 
% William Premerlani and Paul Bizard:
%   see:  https://gentlenav.googlecode.com/files/DCMDraft2.pdf

row_1   = old_gRb(1,:);
row_2   = old_gRb(2,:);

% look at the error associted with row_1 and row_2 they are supposed to be 
% orthogonal, ie: their DOT product should be ZERO
e       = sum( row_1 .* row_2);

% distrubute the error across X and Y
new_row_1 = row_1  - (e/2)*row_2;
new_row_2 = row_2  - (e/2)*row_1;

% compute Z
new_row_3 = cross( new_row_1, new_row_2 );

% normlaize all rows so that their MAG is UNITY
%:  NOTE:  norm([3 4]) is 5
new_row_1 = new_row_1 / norm(new_row_1);
new_row_2 = new_row_2 / norm(new_row_2);
new_row_3 = new_row_3 / norm(new_row_3);

% assemble the NEW gRb matrix
new_gRb = [new_row_1; new_row_2; new_row_3];

end

== matlab function bh_6dof_LIBRARY/MODELS/bh_6DOF_DCM_integrate/Integrate_DCM/MATLAB Function ==
  data: w input; S output
function S = calc_S(w)
%#codegen

x = w(1);
y = w(2);
z = w(3);

S = [    0,  -z,   y;
         z,   0,  -x;
        -y,   x,   0;
    ];

== matlab function bh_6dof_LIBRARY/MODELS/bh_6DOF (Euler Angles)/Calc_DCM/calc_DCM ==
  data: phi input; bRg output; theta input; psi input
function bRg = calc_bRg(phi, theta, psi)
%#codegen

bRg = [ ...
                              cos(phi)*cos(theta),                              cos(theta)*sin(phi),         -sin(theta);
 cos(phi)*sin(psi)*sin(theta) - cos(psi)*sin(phi), cos(phi)*cos(psi) + sin(phi)*sin(psi)*sin(theta), cos(theta)*sin(psi);
 sin(phi)*sin(psi) + cos(phi)*cos(psi)*sin(theta), cos(psi)*sin(phi)*sin(theta) - cos(phi)*sin(psi), cos(psi)*cos(theta);
 ];

end

== matlab function bh_6dof_LIBRARY/MODELS/bh_6DOF_DCM_integrate/Integrate_DCM/MATLAB Function2 ==
  data: bRg input; phi output; theta output; psi output
function [phi, theta, psi] = calc_EUL_angs(bRg)
%#codegen

%NOTE:  this is bRg ... and NOT gRb

% bRg = [ ...
%                               cos(phi)*cos(theta),                              cos(theta)*sin(phi),         -sin(theta);
%  cos(phi)*sin(psi)*sin(theta) - cos(psi)*sin(phi), cos(phi)*cos(psi) + sin(phi)*sin(psi)*sin(theta), cos(theta)*sin(psi);
%  sin(phi)*sin(psi) + cos(phi)*cos(psi)*sin(theta), cos(psi)*sin(phi)*sin(theta) - cos(phi)*sin(psi), cos(psi)*cos(theta);
%  ];

theta = asin( -bRg(1,3) );
phi   = atan2(   bRg(1,2)/cos(theta), bRg(1,1)/cos(theta) ); % <--- SINGULARITY @ theta=pi/2
psi   = atan2(   bRg(2,3)/cos(theta), bRg(3,3)/cos(theta) ); % <--- SINGULARITY @ theta=pi/2
end

== matlab function bh_6dof_LIBRARY/MODELS/bh_6DOF_DCM_integrate/Integrate_DCM/MATLAB Function3 ==
  data: phi input; bRg output; theta input; psi input
function bRg = calc_bRg(phi, theta, psi)
%#codegen

bRg = [ ...
                              cos(phi)*cos(theta),                              cos(theta)*sin(phi),         -sin(theta);
 cos(phi)*sin(psi)*sin(theta) - cos(psi)*sin(phi), cos(phi)*cos(psi) + sin(phi)*sin(psi)*sin(theta), cos(theta)*sin(psi);
 sin(phi)*sin(psi) + cos(phi)*cos(psi)*sin(theta), cos(psi)*sin(phi)*sin(theta) - cos(phi)*sin(psi), cos(psi)*cos(theta);
 ];

end
